simulink model "Model4_Refcalculation1"  (R2023a)
settings: Solver=ode45  StartTime=0.0  StopTime=5  MaxStep=1e-4  RelTol=1e-5  EnableMultiTasking=on
InitFcn:
  | L=0.5e-3
  | R=0.1
  | tau=10e-3
  | f_grid=50
  | Vpeak_d1=150e3
libraries: spsControlledVoltageSourceLib x6, spsCurrentMeasurementLib x3, spsSeriesRLCBranchLib x3, slpidlib x2, powerlib_extras x1, spspowerguiLib x1
settings Model: Creator=Eduardo  LastModifiedBy=citcea
settings SolverCC: AlgebraicLoopSolver=TrustRegion
settings DataIOCC: LimitDataPoints=on  SaveFormat=Array  SignalLoggingSaveFormat=ModelDataLogs  ReturnWorkspaceOutputs=off
settings OptimizationCC: LifeSpan=inf
settings DebuggingCC: SolverPrmCheckMsg=warning  MultiTaskDSMMsg=warning  MultiTaskCondExecSysMsg=none  UnconnectedInputMsg=warning  UnconnectedOutputMsg=warning  UnconnectedLineMsg=warning  StrictBusMsg=ErrorOnBusTreatedAsVector  SFUnexpectedBacktrackingDiag=warning  SFNoUnconditionalDefaultTransitionDiag=warning  SFExecutionAtInitializationDiag=none  ArithmeticOperatorsInVariantConditions=warning
settings HardwareCC: ProdBitPerPointer=32  ProdBitPerSizeT=32  ProdBitPerPtrDiffT=32  ProdLargestAtomicFloat=None  ProdIntDivRoundTo=Undefined  ProdEndianess=Unspecified  ProdWordSize=32  ProdHWDeviceType=32-bit Generic
settings ModelReferenceCC: EnableRefExpFcnMdlSchedulingChecks=on  PropagateSignalLabelsOutOfModel=off
settings SFSimCC: SimUseLocalCustomCode=off  CustomCodeUndefinedFunction=UseInterfaceOnly
settings RTWCC: RTWUseLocalCustomCode=off  DLArmComputeVersion=19.05
settings CodeAppCC: StateflowObjectComments=on
settings GRTTargetCC: TargetLangStandard=C89/C90 (ANSI)
settings ConfigComp: CovMetricSettings=dw  CovSaveCumulativeToWorkspaceVar=on  CovSaveSingleToWorkspaceVar=on  CovExternalEMLEnable=off
settings SimscapeCC: SimscapeNormalizeSystem=off

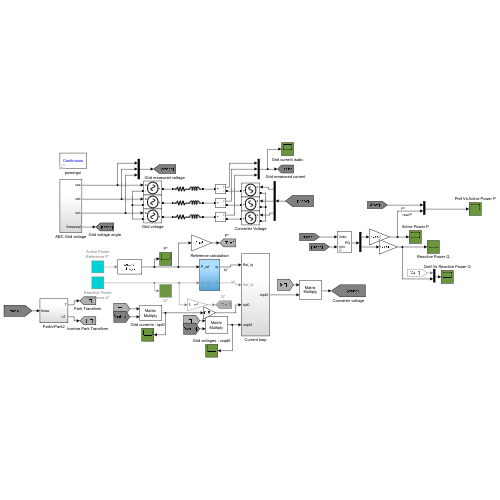
[thumbnail: Simulink's stored preview of the top-level diagram]
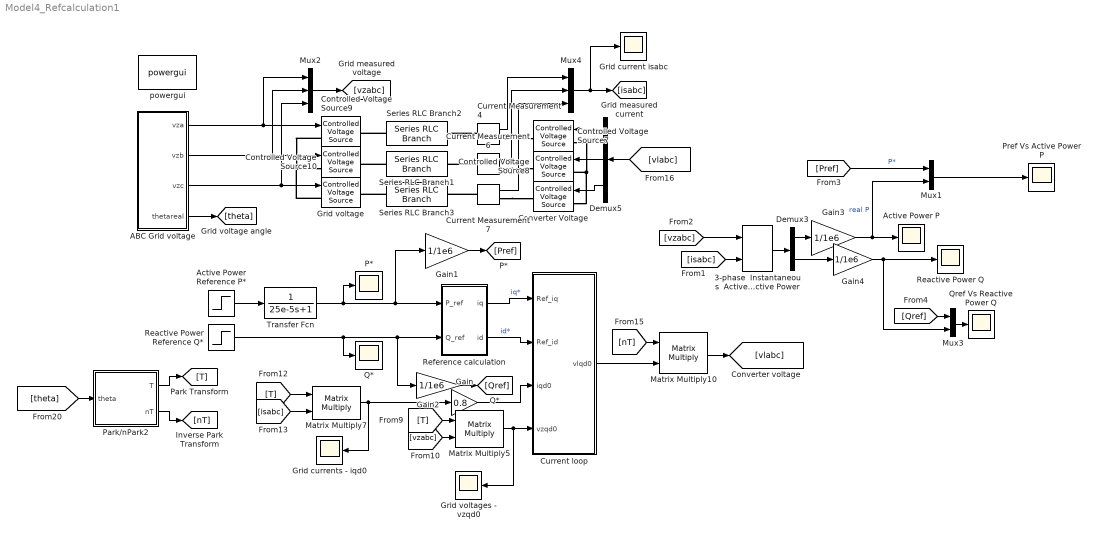
== system Model4_Refcalculation1 ==
  3-phase  Instantaneous  Active & Reactive Power : powerlib_extras/Measurements/3-phase  Instantaneous  Active & Reactive Power
  ABC Grid voltage : Subsystem
  Active Power Reference P* : Step  Time=0.1  After=100e6  SampleTime=0
  Active Power P : Scope
  Controlled Voltage Source{7..10} (4 alike) : spsControlledVoltageSourceLib/Controlled Voltage Source  Initialize=off  Source_Type=AC  Amplitude=0  Phase=0  Frequency=0  Measurements=None
  Converter Voltage : spsControlledVoltageSourceLib/Controlled Voltage Source  Initialize=off  Source_Type=AC  Amplitude=0  Phase=0  Frequency=0  Measurements=None
  Current Measurement4 : spsCurrentMeasurementLib/Current Measurement  PhasorSimulation=off  OutputType=Complex  PSBequivalent=0
  Current Measurement6 : spsCurrentMeasurementLib/Current Measurement  PhasorSimulation=off  OutputType=Complex  PSBequivalent=0
  Current Measurement7 : spsCurrentMeasurementLib/Current Measurement  PhasorSimulation=off  OutputType=Complex  PSBequivalent=0
  Current loop : Subsystem
  Demux3 : Demux  Outputs=2
  Demux5 : Demux  Outputs=3
  Gain : Gain  Gain=0.8
  Gain{1..4} (4 alike) : Gain  Gain=1/1e6
  Grid current isabc : Scope
  Grid currents - iqd0 : Scope
  Grid voltage : spsControlledVoltageSourceLib/Controlled Voltage Source  Initialize=off  Source_Type=AC  Amplitude=0  Phase=0  Frequency=0  Measurements=None
  Grid voltages - vzqd0 : Scope
  Matrix Multiply10 : Product  Multiplication=Matrix(*)
  Matrix Multiply5 : Product  Multiplication=Matrix(*)
  Matrix Multiply7 : Product  Multiplication=Matrix(*)
  Mux1 : Mux  Inputs=2
  Mux2 : Mux  Inputs=3
  Mux3 : Mux  Inputs=2
  Mux4 : Mux  Inputs=3
  P* : Scope
  Park/nPark2 : Subsystem
  Pref Vs Active Power P : Scope
  Q* : Scope
  Qref Vs Reactive Power Q : Scope
  Reactive Power Reference Q* : Step  Time=0.3  After=10e6  SampleTime=0
  Reactive Power Q : Scope
  Reference calculation : Subsystem
  Series RLC Branch1 : spsSeriesRLCBranchLib/Series RLC Branch  LConnTagsString=__new0  RConnTagsString=__new0  BranchType=RL  Resistance=R  Inductance=L  SetiL0=off  InitialCurrent=0  Capacitance=0  Setx0=off  InitialVoltage=0  Measurements=None
  Series RLC Branch2 : spsSeriesRLCBranchLib/Series RLC Branch  LConnTagsString=__new0  RConnTagsString=__new0  BranchType=RL  Resistance=R  Inductance=L  SetiL0=off  InitialCurrent=0  Capacitance=0  Setx0=off  InitialVoltage=0  Measurements=None
  Series RLC Branch3 : spsSeriesRLCBranchLib/Series RLC Branch  LConnTagsString=__new0  RConnTagsString=__new0  BranchType=RL  Resistance=R  Inductance=L  SetiL0=off  InitialCurrent=0  Capacitance=0  Setx0=off  InitialVoltage=0  Measurements=None
  Transfer Fcn : TransferFcn  Denominator=[25e-5 1]
  powergui : spspowerguiLib/powergui  Priority=1  SimulationMode=Continuous  SampleTime=50e-6  frequency=60  Iterations=50  frequencyindice=0  Pbase=100e6  ErrMax=1e-4  UnitsV=kV  UnitsW=MW  buscounter=0  FunctionMessages=off  echomessages=off  EnableUseOfTLC=off  CurrentSourceSwitches=on  DisableSnubberDevices=off  DisableRonSwitches=off  DisableVfSwitches=off  DisplayEquations=off  AutomaticDiscreteSolvers=off  SolverType=Tustin  Interpol=off  ExternalGateDelay=off  methode=off  Ts=0  x0status=blocks  SPID=off  SwTol=0  HookPort=off  NonlinearTolerance=1e-4  nMaxIteration=100  ContinueOnMaxIteration=off  RestoreLinks=warning  ResistiveCurrentMeasurement=off  Frange=[0:2:500]  Ylog=off  Xlog=on  ShowGrid=off  save=off  variable=ZData  structure=0  ZoomFFT=off  StartTime=0.0  cycles=1  DisplayStyle=1  fundamental=60  FreqAxis=off  MaxFrequency=1000  frequencyindicesteady=1  RmsSteady=1  display=off
  wires:
  Mux2/1 -> [vzabc]
  Mux4/1 -> Grid current isabc/1, [isabc]
  ABC Grid voltage/4(thetareal) -> [theta]
  Matrix Multiply7/1 -> Gain/1, Grid currents - iqd0/1
  [T] -> Matrix Multiply7/1
  [isabc] -> Matrix Multiply7/2
  Demux5/1 -> Controlled Voltage Source7/1
  Demux5/2 -> Controlled Voltage Source8/1
  Demux5/3 -> Converter Voltage/1
  ABC Grid voltage/1(vza) -> Controlled Voltage Source9/1, Mux2/1
  ABC Grid voltage/2(vzb) -> Controlled Voltage Source10/1, Mux2/2
  ABC Grid voltage/3(vzc) -> Grid voltage/1, Mux2/3
  Park/nPark2/1(T) -> [T]
  [theta] -> Park/nPark2/1(theta)
  [vlabc] -> Demux5/1
  Park/nPark2/2("nT ") -> [nT]
  Current Measurement4/1 -> Mux4/1
  Current Measurement6/1 -> Mux4/2
  Current Measurement7/1 -> Mux4/3
  Reference calculation/1(iq) -> Current loop/1(Ref_iq)  "iq*"
  Reference calculation/2(id) -> Current loop/2(Ref_id)  "id*"
  Current loop/1(vlqd0) -> Matrix Multiply10/2
  [T] -> Matrix Multiply5/1
  [vzabc] -> Matrix Multiply5/2
  Matrix Multiply5/1 -> Grid voltages - vzqd0/1, Current loop/4(vzqd0)
  [nT] -> Matrix Multiply10/1
  Matrix Multiply10/1 -> [vlabc]
  Active Power Reference P*/1 -> Transfer Fcn/1
  [isabc] -> 3-phase  Instantaneous  Active & Reactive Power/2
  [vzabc] -> 3-phase  Instantaneous  Active & Reactive Power/1
  Demux3/1 -> Gain3/1
  Demux3/2 -> Gain4/1
  3-phase  Instantaneous  Active & Reactive Power/1 -> Demux3/1
  Mux1/1 -> Pref Vs Active Power P/1
  [Pref] -> Mux1/1  "P*"
  Gain3/1 -> Mux1/2, Active Power P/1  "real P"
  Mux3/1 -> Qref Vs Reactive Power Q/1
  [Qref] -> Mux3/1
  Gain4/1 -> Mux3/2, Reactive Power Q/1
  Gain1/1 -> [Pref]
  Reactive Power Reference Q*/1 -> Gain2/1, Reference calculation/2(Q_ref), Q*/1
  Gain2/1 -> [Qref]
  Transfer Fcn/1 -> P*/1, Reference calculation/1(P_ref), Gain1/1
  Gain/1 -> Current loop/3(iqd0)
  connections:
  Controlled Voltage Source9/LConn1 -- Controlled Voltage Source10/LConn1 -- Grid voltage/LConn1
  Controlled Voltage Source7/LConn1 -- Controlled Voltage Source8/LConn1 -- Converter Voltage/LConn1
  Current Measurement6/RConn1 -- Controlled Voltage Source8/RConn1
  Current Measurement7/RConn1 -- Converter Voltage/RConn1
  Current Measurement4/LConn1 -- Series RLC Branch2/RConn1
  Series RLC Branch2/LConn1 -- Controlled Voltage Source9/RConn1
  Current Measurement7/LConn1 -- Series RLC Branch3/RConn1
  Current Measurement6/LConn1 -- Series RLC Branch1/RConn1
  Series RLC Branch3/LConn1 -- Grid voltage/RConn1
  Current Measurement4/RConn1 -- Controlled Voltage Source7/RConn1
  Series RLC Branch1/LConn1 -- Controlled Voltage Source10/RConn1

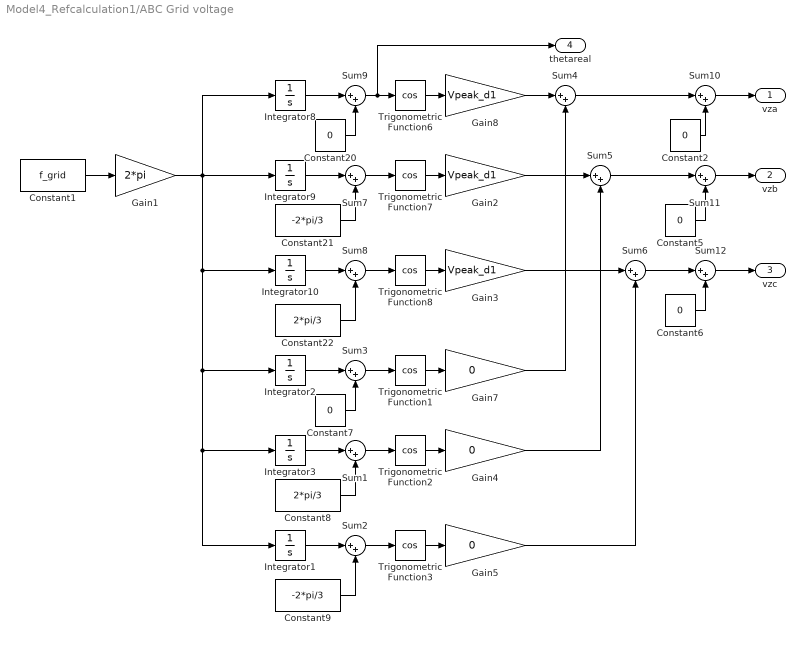
== system Model4_Refcalculation1/ABC Grid voltage ==
  Constant1 : Constant  Value=f_grid
  Constant{2,5..7,20} (5 alike) : Constant  Value=0
  Constant21 : Constant  Value=-2*pi/3
  Constant22 : Constant  Value=2*pi/3
  Constant8 : Constant  Value=2*pi/3
  Constant9 : Constant  Value=-2*pi/3
  Gain1 : Gain  Gain=2*pi
  Gain2 : Gain  Gain=Vpeak_d1
  Gain3 : Gain  Gain=Vpeak_d1
  Gain4 : Gain  Gain=0
  Gain5 : Gain  Gain=0
  Gain7 : Gain  Gain=0
  Gain8 : Gain  Gain=Vpeak_d1
  Integrator{1..3,8..10} (6 alike) : Integrator
  Sum{1..12} (12 alike) : Sum  Inputs=|++
  Trigonometric Function{1..3,6..8} (6 alike) : Trigonometry  Operator=cos
  vza : Outport
  vzb : Outport  Port=2
  vzc : Outport  Port=3
  thetareal : Outport  Port=4
  wires:
  Sum12/1 -> vzc/1
  Sum11/1 -> vzb/1
  Sum10/1 -> vza/1
  Constant6/1 -> Sum12/2
  Constant5/1 -> Sum11/2
  Constant2/1 -> Sum10/2
  Sum6/1 -> Sum12/1
  Sum5/1 -> Sum11/1
  Sum4/1 -> Sum10/1
  Gain5/1 -> Sum6/2
  Gain4/1 -> Sum5/2
  Gain7/1 -> Sum4/2
  Trigonometric Function2/1 -> Gain4/1
  Trigonometric Function3/1 -> Gain5/1
  Sum3/1 -> Trigonometric Function1/1
  Constant9/1 -> Sum2/2
  Integrator1/1 -> Sum2/1
  Constant8/1 -> Sum1/2
  Integrator2/1 -> Sum3/1
  Gain1/1 -> Integrator9/1, Integrator8/1, Integrator10/1, Integrator2/1, Integrator1/1, Integrator3/1
  Sum1/1 -> Trigonometric Function2/1
  Constant7/1 -> Sum3/2
  Trigonometric Function1/1 -> Gain7/1
  Integrator3/1 -> Sum1/1
  Sum2/1 -> Trigonometric Function3/1
  Gain3/1 -> Sum6/1
  Gain2/1 -> Sum5/1
  Gain8/1 -> Sum4/1
  Trigonometric Function7/1 -> Gain2/1
  Trigonometric Function8/1 -> Gain3/1
  Constant1/1 -> Gain1/1
  Sum9/1 -> thetareal/1, Trigonometric Function6/1
  Constant22/1 -> Sum8/2
  Integrator10/1 -> Sum8/1
  Constant21/1 -> Sum7/2
  Integrator8/1 -> Sum9/1
  Sum7/1 -> Trigonometric Function7/1
  Constant20/1 -> Sum9/2
  Trigonometric Function6/1 -> Gain8/1
  Integrator9/1 -> Sum7/1
  Sum8/1 -> Trigonometric Function8/1

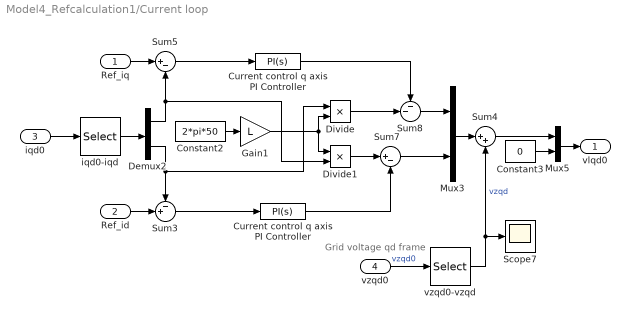
== system Model4_Refcalculation1/Current loop ==
  note: Grid voltage qd frame
  Ref_iq : Inport
  Ref_id : Inport  Port=2
  iqd0 : Inport  Port=3
  vzqd0 : Inport  Port=4
  Constant2 : Constant  Value=2*pi*50  SampleTime=-1
  Constant3 : Constant  Value=0
  Current control q axis PI Controller : slpidlib/PID Controller  Controller=PI  Form=Parallel  TimeDomain=Continuous-time  UseExternalTs=off  SampleTime=1  IntegratorMethod=Forward Euler  FilterMethod=Forward Euler  ControllerParametersSource=internal  P=L/tau  I=R/tau  UseKiTs=off  D=0  N=100  UseFilter=on  TunerSelectOption=Transfer Function Based (PID Tuner App)  InitialConditionSource=internal  InitialConditionForIntegrator=0  InitialConditionForFilter=0  DifferentiatorICPrevScaledInput=0  ExternalReset=none  TrackingMode=off  Kt=1  LimitOutput=off  SatLimitsSource=internal  UpperSaturationLimit=inf  LowerSaturationLimit=-inf  LinearizeAsGain=on  AntiWindupMode=none  Kb=1  LimitIntegrator=off  UpperIntegratorSaturationLimit=inf  LowerIntegratorSaturationLimit=-inf  POutMin=[]  POutMax=[]  IOutMin=[]  IOutMax=[]  DOutMin=[]  DOutMax=[]  NOutMin=[]  NOutMax=[]  SumOutMin=[]  SumOutMax=[]  SaturationOutMin=[]  SaturationOutMax=[]  PParamMin=[]  PParamMax=[]  IParamMin=[]  IParamMax=[]  DParamMin=[]  DParamMax=[]  NParamMin=[]  NParamMax=[]  KbParamMin=[]  KbParamMax=[]  KtParamMin=[]  KtParamMax=[]  KbOutMin=[]  KbOutMax=[]  KtOutMin=[]  KtOutMax=[]  IntegratorOutMin=[]  IntegratorOutMax=[]  FilterOutMin=[]  FilterOutMax=[]  SumI1OutMin=[]  SumI1OutMax=[]  SumI2OutMin=[]  SumI2OutMax=[]  SumI3OutMin=[]  SumI3OutMax=[]  SumI4OutMin=[]  SumI4OutMax=[]  SumDOutMin=[]  SumDOutMax=[]  DifferentiatorOutMin=[]  DifferentiatorOutMax=[]  FilterDiffOutCoefMin=[]  FilterDiffOutCoefMax=[]  ReciprocalOutMin=[]  ReciprocalOutMax=[]  SumDenOutMin=[]  SumDenOutMax=[]  SumNumOutMin=[]  SumNumOutMax=[]  DivideOutMin=[]  DivideOutMax=[]  UdiffTsProdOutMin=[]  UdiffTsProdOutMax=[]  NTsProdOutMin=[]  NTsProdOutMax=[]  UintegralTsProdOutMin=[]  UintegralTsProdOutMax=[]  UngainTsProdOutMin=[]  UngainTsProdOutMax=[]  ClampingZeroOutDataTypeStr=Inherit: Inherit via back propagation  ClampingZeroOutMin=[]  ClampingZeroOutMax=[]  FilterDenConstantOutDataTypeStr=Inherit: Inherit via back propagation  FilterDenConstantOutMin=[]  FilterDenConstantOutMax=[]  PCopyOutDataTypeStr=Inherit: Inherit via back propagation  PCopyOutMin=[]  PCopyOutMax=[]  NCopyOutDataTypeStr=Inherit: Inherit via back propagation  NCopyOutMin=[]  NCopyOutMax=[]  IntegratorContinuousStateAttributes=''  IntegratorStateMustResolveToSignalObject=off  IntegratorRTWStateStorageClass=Auto  FilterContinuousStateAttributes=''  FilterStateMustResolveToSignalObject=off  FilterRTWStateStorageClass=Auto  ParallelPVariant=InternalParameters  IdealPVariant=Disabled  IVariant=InternalParameters  DVariant=Disabled  IntegratorVariant=Continuous  SatVariant=Disabled  AWVariant=Passthrough  PCopyVariant=Disabled  TRVariant=Disabled  FdbkBlocksVariant=Forward  IdealPFdbkVariant=Disabled  SatFdbkVariant=Disabled  DerivativeFilterVariant=Disabled  NVariant=Disabled  NCopyVariant=Disabled_SignalSpec  FilterICVariant=Disabled  IntegratorICVariant=InternalICs  ExternalResetVariant=Disabled  TRSumVariant=Passthrough  SumFdbkVariant=Disabled  SumVariant=Sum_PI  TsampFilterVariant=InternalTs  TsampNgainVariant=Passthrough  TsampIntegralVariant=Disabled_SignalSpec  ExternalSaturationOutDataTypeStr=Inherit: Same as second input
  "Current control q axis PI Controller " : slpidlib/PID Controller  Controller=PI  Form=Parallel  TimeDomain=Continuous-time  UseExternalTs=off  SampleTime=1  IntegratorMethod=Forward Euler  FilterMethod=Forward Euler  ControllerParametersSource=internal  P=L/tau  I=R/tau  UseKiTs=off  D=0  N=100  UseFilter=on  TunerSelectOption=Transfer Function Based (PID Tuner App)  InitialConditionSource=internal  InitialConditionForIntegrator=0  InitialConditionForFilter=0  DifferentiatorICPrevScaledInput=0  ExternalReset=none  TrackingMode=off  Kt=1  LimitOutput=off  SatLimitsSource=internal  UpperSaturationLimit=inf  LowerSaturationLimit=-inf  LinearizeAsGain=on  AntiWindupMode=none  Kb=1  LimitIntegrator=off  UpperIntegratorSaturationLimit=inf  LowerIntegratorSaturationLimit=-inf  POutMin=[]  POutMax=[]  IOutMin=[]  IOutMax=[]  DOutMin=[]  DOutMax=[]  NOutMin=[]  NOutMax=[]  SumOutMin=[]  SumOutMax=[]  SaturationOutMin=[]  SaturationOutMax=[]  PParamMin=[]  PParamMax=[]  IParamMin=[]  IParamMax=[]  DParamMin=[]  DParamMax=[]  NParamMin=[]  NParamMax=[]  KbParamMin=[]  KbParamMax=[]  KtParamMin=[]  KtParamMax=[]  KbOutMin=[]  KbOutMax=[]  KtOutMin=[]  KtOutMax=[]  IntegratorOutMin=[]  IntegratorOutMax=[]  FilterOutMin=[]  FilterOutMax=[]  SumI1OutMin=[]  SumI1OutMax=[]  SumI2OutMin=[]  SumI2OutMax=[]  SumI3OutMin=[]  SumI3OutMax=[]  SumI4OutMin=[]  SumI4OutMax=[]  SumDOutMin=[]  SumDOutMax=[]  DifferentiatorOutMin=[]  DifferentiatorOutMax=[]  FilterDiffOutCoefMin=[]  FilterDiffOutCoefMax=[]  ReciprocalOutMin=[]  ReciprocalOutMax=[]  SumDenOutMin=[]  SumDenOutMax=[]  SumNumOutMin=[]  SumNumOutMax=[]  DivideOutMin=[]  DivideOutMax=[]  UdiffTsProdOutMin=[]  UdiffTsProdOutMax=[]  NTsProdOutMin=[]  NTsProdOutMax=[]  UintegralTsProdOutMin=[]  UintegralTsProdOutMax=[]  UngainTsProdOutMin=[]  UngainTsProdOutMax=[]  ClampingZeroOutDataTypeStr=Inherit: Inherit via back propagation  ClampingZeroOutMin=[]  ClampingZeroOutMax=[]  FilterDenConstantOutDataTypeStr=Inherit: Inherit via back propagation  FilterDenConstantOutMin=[]  FilterDenConstantOutMax=[]  PCopyOutDataTypeStr=Inherit: Inherit via back propagation  PCopyOutMin=[]  PCopyOutMax=[]  NCopyOutDataTypeStr=Inherit: Inherit via back propagation  NCopyOutMin=[]  NCopyOutMax=[]  IntegratorContinuousStateAttributes=''  IntegratorStateMustResolveToSignalObject=off  IntegratorRTWStateStorageClass=Auto  FilterContinuousStateAttributes=''  FilterStateMustResolveToSignalObject=off  FilterRTWStateStorageClass=Auto  ParallelPVariant=InternalParameters  IdealPVariant=Disabled  IVariant=InternalParameters  DVariant=Disabled  IntegratorVariant=Continuous  SatVariant=Disabled  AWVariant=Passthrough  PCopyVariant=Disabled  TRVariant=Disabled  FdbkBlocksVariant=Forward  IdealPFdbkVariant=Disabled  SatFdbkVariant=Disabled  DerivativeFilterVariant=Disabled  NVariant=Disabled  NCopyVariant=Disabled_SignalSpec  FilterICVariant=Disabled  IntegratorICVariant=InternalICs  ExternalResetVariant=Disabled  TRSumVariant=Passthrough  SumFdbkVariant=Disabled  SumVariant=Sum_PI  TsampFilterVariant=InternalTs  TsampNgainVariant=Passthrough  TsampIntegralVariant=Disabled_SignalSpec  ExternalSaturationOutDataTypeStr=Inherit: Same as second input
  Demux2 : Demux  Outputs=2
  Divide : Product  Inputs=**
  Divide1 : Product  Inputs=**
  Gain1 : Gain  Gain=L
  Mux3 : Mux  Inputs=2
  Mux5 : Mux  Inputs=2
  Scope7 : Scope
  Sum3 : Sum  Inputs=-+|
  Sum4 : Sum  Inputs=|++
  Sum5 : Sum  Inputs=|+-
  Sum7 : Sum  Inputs=|+-
  Sum8 : Sum  Inputs=--|
  iqd0-iqd : Selector  InputPortWidth=3  IndexOptions=Index vector (dialog)  Indices=[1 2]  OutputSizes=1
  vzqd0-vzqd : Selector  InputPortWidth=3  IndexOptions=Index vector (dialog)  Indices=[1 2]  OutputSizes=1
  vlqd0 : Outport
  wires:
  Ref_iq/1 -> Sum5/1
  Ref_id/1 -> Sum3/2
  Current control q axis PI Controller/1 -> Sum8/1
  Mux3/1 -> Sum4/1
  vzqd0-vzqd/1 -> Scope7/1, Sum4/2  "vzqd"
  Sum5/1 -> Current control q axis PI Controller/1
  Gain1/1 -> Divide1/1, Divide/2
  Constant2/1 -> Gain1/1
  Demux2/1 -> Divide1/2, Sum5/2
  Divide/1 -> Sum8/2
  vzqd0/1 -> vzqd0-vzqd/1  "vzqd0"
  Mux5/1 -> vlqd0/1
  Sum4/1 -> Mux5/1
  Sum7/1 -> Mux3/2
  Sum3/1 -> "Current control q axis PI Controller "/1
  Divide1/1 -> Sum7/1
  Sum8/1 -> Mux3/1
  "Current control q axis PI Controller "/1 -> Sum7/2
  Constant3/1 -> Mux5/2
  Demux2/2 -> Sum3/1, Divide/1
  iqd0/1 -> iqd0-iqd/1
  iqd0-iqd/1 -> Demux2/1

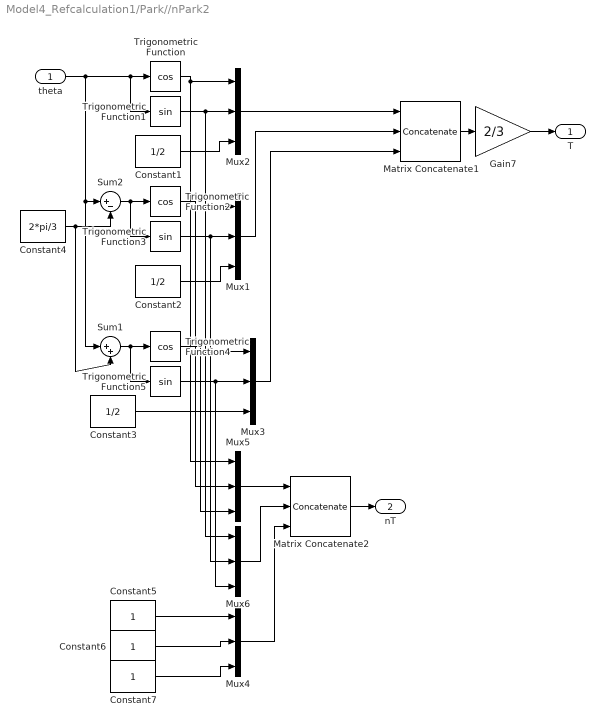
== system Model4_Refcalculation1/Park//nPark2 ==
  theta : Inport
  Constant1 : Constant  Value=1/2  SampleTime=0
  Constant2 : Constant  Value=1/2  SampleTime=0
  Constant3 : Constant  Value=1/2  SampleTime=0
  Constant4 : Constant  Value=2*pi/3  SampleTime=0
  Constant5 : Constant  SampleTime=0
  Constant6 : Constant  SampleTime=0
  Constant7 : Constant  SampleTime=0
  Gain7 : Gain  Gain=2/3
  Matrix Concatenate1 : Concatenate  NumInputs=3  Mode=Multidimensional array  ConcatenateDimension=2
  Matrix Concatenate2 : Concatenate  NumInputs=3  Mode=Multidimensional array  ConcatenateDimension=2
  Mux{1..6} (6 alike) : Mux  Inputs=3
  Sum1 : Sum  Inputs=|++
  Sum2 : Sum  Inputs=|+-
  Trigonometric Function : Trigonometry  Operator=cos
  Trigonometric Function1 : Trigonometry
  Trigonometric Function2 : Trigonometry  Operator=cos
  Trigonometric Function3 : Trigonometry
  Trigonometric Function4 : Trigonometry  Operator=cos
  Trigonometric Function5 : Trigonometry
  T : Outport
  "nT " : Outport  Port=2
  wires:
  Matrix Concatenate2/1 -> "nT "/1
  Gain7/1 -> T/1
  theta/1 -> Trigonometric Function1/1, Trigonometric Function/1, Sum2/1, Sum1/1
  Mux6/1 -> Matrix Concatenate2/2
  Mux5/1 -> Matrix Concatenate2/1
  Matrix Concatenate1/1 -> Gain7/1
  Mux3/1 -> Matrix Concatenate1/3
  Mux1/1 -> Matrix Concatenate1/2
  Mux2/1 -> Matrix Concatenate1/1
  Trigonometric Function5/1 -> Mux3/2, Mux6/3
  Trigonometric Function4/1 -> Mux5/3, Mux3/1
  Trigonometric Function3/1 -> Mux1/2, Mux6/2
  Trigonometric Function2/1 -> Mux1/1, Mux5/2
  Trigonometric Function1/1 -> Mux6/1, Mux2/2
  Trigonometric Function/1 -> Mux5/1, Mux2/1
  Constant4/1 -> Sum1/2, Sum2/2
  Sum1/1 -> Trigonometric Function5/1, Trigonometric Function4/1
  Sum2/1 -> Trigonometric Function3/1, Trigonometric Function2/1
  Constant1/1 -> Mux2/3
  Constant2/1 -> Mux1/3
  Constant3/1 -> Mux3/3
  Constant5/1 -> Mux4/1
  Constant6/1 -> Mux4/2
  Constant7/1 -> Mux4/3
  Mux4/1 -> Matrix Concatenate2/3

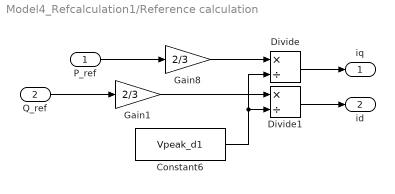
== system Model4_Refcalculation1/Reference calculation ==
  P_ref : Inport
  Q_ref : Inport  Port=2
  Constant6 : Constant  Value=Vpeak_d1
  Divide : Product  Inputs=*/
  Divide1 : Product  Inputs=*/
  Gain1 : Gain  Gain=2/3
  Gain8 : Gain  Gain=2/3
  iq : Outport
  id : Outport  Port=2
  wires:
  P_ref/1 -> Gain8/1
  Q_ref/1 -> Gain1/1
  Gain8/1 -> Divide/1
  Gain1/1 -> Divide1/1
  Constant6/1 -> Divide1/2, Divide/2
  Divide1/1 -> id/1
  Divide/1 -> iq/1
